simulink model "simulink_model_advanced_closed_loop"  (R2019a)
settings: Solver=VariableStepAuto  StartTime=0.0  StopTime=2  RelTol=1e-3
settings Model: Creator=oj  LastModifiedBy=oj

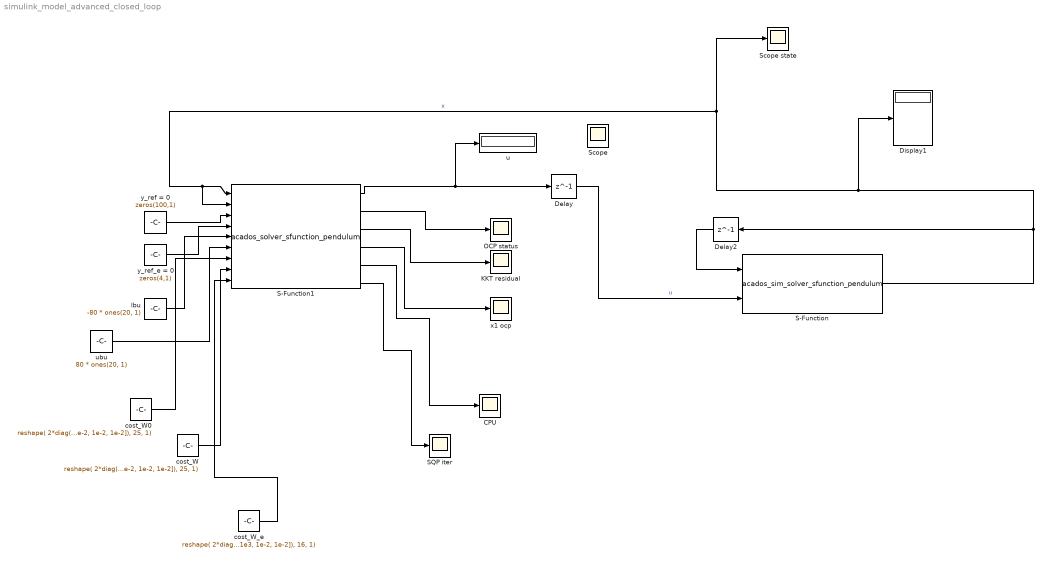
== system simulink_model_advanced_closed_loop ==
  CPU : Scope
      settings: Description=status
  Delay : Delay  DelayLength=1  InitialCondition=0
  Delay2 : Delay  DelayLength=1  InitialCondition=[1 pi 0 0]
  Display1 : Display
  KKT residual : Scope
      settings: Description=status
  OCP status : Scope
      settings: Description=status
  S-Function : S-Function  FunctionName=acados_sim_solver_sfunction_pendulum  SFunctionDeploymentMode=off  EnableBusSupport=off
  S-Function1 : S-Function  FunctionName=acados_solver_sfunction_pendulum  SFunctionDeploymentMode=off  EnableBusSupport=off
  SQP iter : Scope
      settings: Description=status
  Scope state : Scope
  cost_W : Constant  Value=reshape( 2*diag([1e3, 1e3, 1e-2, 1e-2, 1e-2]), 25, 1)
  cost_W0 : Constant  Value=reshape( 2*diag([1e3, 1e3, 1e-2, 1e-2, 1e-2]), 25, 1)
  cost_W_e : Constant  Value=reshape( 2*diag([1e3, 1e3, 1e-2, 1e-2]), 16, 1)
  lbu : Constant  Value=-80 * ones(20, 1)
  u : Display
  ubu : Constant  Value=80 * ones(20, 1)
  x1 ocp : Scope
      settings: Description=status
  y_ref = 0 : Constant  Value=zeros(100,1)
  y_ref_e = 0 : Constant  Value=zeros(4,1)
  Scope : Scope
  wires:
  S-Function/1 -> Display1/1, Scope state/1, S-Function1/2, S-Function1/1, Delay2/1  "x"
  S-Function1/1 -> u/1, Delay/1
  S-Function1/2 -> OCP status/1
  S-Function1/3 -> KKT residual/1
  S-Function1/4 -> x1 ocp/1
  S-Function1/5 -> CPU/1
  y_ref = 0/1 -> S-Function1/3
  y_ref_e = 0/1 -> S-Function1/4
  lbu/1 -> S-Function1/5
  ubu/1 -> S-Function1/6
  Delay/1 -> S-Function/2  "u"
  Delay2/1 -> S-Function/1
  S-Function1/6 -> SQP iter/1
  cost_W0/1 -> S-Function1/7
  cost_W/1 -> S-Function1/8
  cost_W_e/1 -> S-Function1/9
